simulink model "planta_CODESYS"  (R2025b)
settings: Solver=FixedStepAuto  StartTime=0.0  StopTime=inf  FixedStep=Ts2  MaxStep=1e-3  RelTol=1e-3
undefined symbols (not defined in the file): ah_max, at_max, bcx, bcy, bh_eq, bhb, bhEb, bhwu, bt, bt_eq, btb, btw, g, Hc, ih, it, Jh_eq, Jt_eq, Kcy, khwu, Ki_h, Ki_t, Kp_h, Kp_t, Ktw, lambda, Lh, Lh0, lh_0, Lt, magnitude, Mc_max, Ms, Mt, rhd, rtd, tau_hm, tau_tm, Thb_Max, ThEb_Max, Thm_0, Thm_Max, titahm_0, titatm_0, Ts0, Ts1, Ts2, Ttb_Max, Ttm_0, Ttm_Max, vh_0, vlx_0, vly_0, vt_0, vt_max, Wc, whm_0, whm_rated, wtm_0, xl_0 ... (+9)
libraries: simulink x10, opcualib x9, simulink_extras x2, dspnetwork x2, sl3dlib x1, hostiolib x1
(part 2 of 2)

== system planta_CODESYS/Controlador Izaje2 ==
  seleccion : Inport
  yh_enc : Inport  Port=2
  m_est : Inport  Port=3
  vh_lim : Inport  Port=4
  BRK_h : Inport  Port=5
  BRK_hE : Inport  Port=6
  vy_cmd : Inport  Port=7
  AND : Logic  IconShape=distinctive  AllPortsSameDT=off  OutDataTypeStr=boolean
  Controlador de Velocidad : MATLAB Function  TreatAsAtomicUnit=on
  Delay One Step : Delay  DelayLength=1  InitialCondition=Thm_0
  Modulación de la Referencia : MATLAB Function  TreatAsAtomicUnit=on
  Observador de Estado : MATLAB Function  TreatAsAtomicUnit=on
  vh_obs : Outport
  Thm_ref : Outport  Port=2
  wires:
  seleccion/1 -> Modulación de la Referencia/2(seleccion)
  m_est/1 -> Controlador de Velocidad/1(m_est)
  Delay One Step/1 -> Observador de Estado/2(Thm_ref)
  yh_enc/1 -> Observador de Estado/1(yh_enc)
  Observador de Estado/1(vh_obs) -> Controlador de Velocidad/3(vh_obs), vh_obs/1
  vy_cmd/1 -> Modulación de la Referencia/1(vy_cmd)
  Modulación de la Referencia/1(vh_ref) -> Controlador de Velocidad/2(vh_ref)
  AND/1 -> Controlador de Velocidad/4(BRK)
  BRK_hE/1 -> AND/2
  vh_lim/1 -> Modulación de la Referencia/3(vh_lim)
  BRK_h/1 -> AND/1
  Controlador de Velocidad/1(Thm_ref) -> Delay One Step/1, Thm_ref/1

== system planta_CODESYS/Modulador Carro ==
  Ttm_ref : Inport
  BRK_t : Inport  Port=2
  Constant1 : Constant  Value=0
  Gain2 : Gain  Gain=1/tau_tm
  Integrator : Integrator  InitialCondition=Ttm_0
  Saturation : Saturate  UpperLimit=Ttm_Max  LowerLimit=-Ttm_Max
  Sum : Sum  Inputs=|+-
  Switch : Switch  Criteria=u2 > Threshold  SaturateOnIntegerOverflow=off  InputSameDT=off
  Ttm : Outport
  wires:
  Saturation/1 -> Sum/1  "Ttm_lim"
  Sum/1 -> Gain2/1
  Gain2/1 -> Integrator/1
  Integrator/1 -> Ttm/1, Sum/2
  Ttm_ref/1 -> Switch/1
  BRK_t/1 -> Switch/2
  Switch/1 -> Saturation/1
  Constant1/1 -> Switch/3

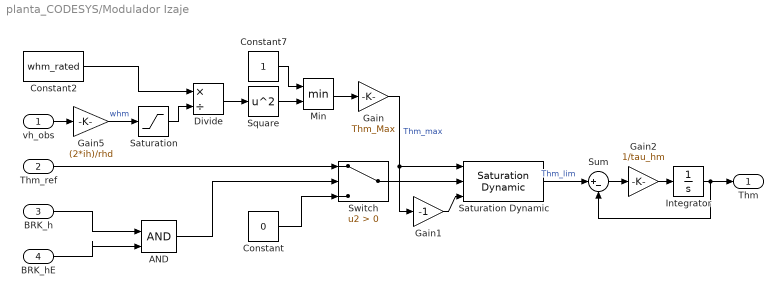
== system planta_CODESYS/Modulador Izaje ==
  vh_obs : Inport
  Thm_ref : Inport  Port=2
  BRK_h : Inport  Port=3
  BRK_hE : Inport  Port=4
  AND : Logic  IconShape=distinctive  AllPortsSameDT=off  OutDataTypeStr=boolean
  Constant : Constant  Value=0
  Constant2 : Constant  Value=whm_rated
  Constant7 : Constant
  Divide : Product  Inputs=*/
  Gain : Gain  Gain=Thm_Max
  Gain1 : Gain  Gain=-1
  Gain2 : Gain  Gain=1/tau_hm
  Gain5 : Gain  Gain=(2*ih)/rhd
  Integrator : Integrator  InitialCondition=Thm_0
  Min : MinMax  Inputs=2
  Saturation : Saturate  UpperLimit=inf  LowerLimit=whm_rated
  Saturation Dynamic : simulink/Discontinuities/Saturation Dynamic  OutMin=[]  OutMax=[]  OutDataTypeStr=Inherit: Same as second input  OutDataType=fixdt(1, 16)  OutScaling=2^-10  DoSatur=off
  Square : Math  Operator=square
  Sum : Sum  Inputs=|+-
  Switch : Switch  Criteria=u2 > Threshold  SaturateOnIntegerOverflow=off  InputSameDT=off
  Thm : Outport
  wires:
  Constant2/1 -> Divide/1
  Min/1 -> Gain/1
  Constant7/1 -> Min/1
  Gain/1 -> Gain1/1, Saturation Dynamic/1  "Thm_max"
  Saturation/1 -> Divide/2
  Square/1 -> Min/2
  Divide/1 -> Square/1
  vh_obs/1 -> Gain5/1
  Gain1/1 -> Saturation Dynamic/3
  Saturation Dynamic/1 -> Sum/1  "Thm_lim"
  Sum/1 -> Gain2/1
  Gain2/1 -> Integrator/1
  Integrator/1 -> Thm/1, Sum/2
  Thm_ref/1 -> Switch/1
  BRK_h/1 -> AND/1
  Switch/1 -> Saturation Dynamic/2
  BRK_hE/1 -> AND/2
  AND/1 -> Switch/2
  Gain5/1 -> Saturation/1  "whm"
  Constant/1 -> Switch/3

== system planta_CODESYS/Sensores Carro ==
  θtm : Inport
  xt : Inport  Port=2
  Encoder Carro : Subsystem
  Fines de carrera carro (rieles) : Subsystem
  xtd_enc : Outport
  FCE_izquierdo : Outport  Port=2
  FCE_derecho : Outport  Port=3
  FC_izquierdo : Outport  Port=4
  FC_derecho : Outport  Port=5
  wires:
  Fines de carrera carro (rieles)/1(FC_derecho) -> FC_derecho/1
  θtm/1 -> Encoder Carro/1(θtm)
  Fines de carrera carro (rieles)/2(FC_izquierdo) -> FC_izquierdo/1
  Fines de carrera carro (rieles)/3(FCE_derecho) -> FCE_derecho/1
  Fines de carrera carro (rieles)/4(FCE_izquierdo) -> FCE_izquierdo/1
  xt/1 -> Fines de carrera carro (rieles)/1(xt)
  Encoder Carro/1(xtd_enc) -> xtd_enc/1

== system planta_CODESYS/Sensores Izaje ==
  θhm : Inport
  Encoder Izaje : Subsystem
  Fines de carrera izaje (tambor) : Subsystem
  yh_enc : Outport
  FCE_inferior : Outport  Port=2
  FCE_superior : Outport  Port=3
  FC_inferior : Outport  Port=4
  FC_superior : Outport  Port=5
  wires:
  Fines de carrera izaje (tambor)/1(FC_superior) -> FC_superior/1
  Fines de carrera izaje (tambor)/4(FCE_inferior) -> FCE_inferior/1
  Fines de carrera izaje (tambor)/2(FC_inferior) -> FC_inferior/1
  Encoder Izaje/1(yh_enc) -> Fines de carrera izaje (tambor)/1(y_enc), yh_enc/1
  θhm/1 -> Encoder Izaje/1(θhm)
  Fines de carrera izaje (tambor)/3(FCE_superior) -> FCE_superior/1

== system planta_CODESYS/Subsistema Carro ==
  Fhw : Inport
  θl : Inport  Port=2
  Ttm : Inport  Port=3
  BRK_t : Inport  Port=4
  Accionamiento carro : Subsystem
  Dinámica carro : Subsystem
  Fuerza cable carro : Subsystem
  at : Outport
  vt : Outport  Port=2
  xt : Outport  Port=3
  θtm : Outport  Port=4
  wires:
  [Ftw] -> Accionamiento carro/1(Ftw)
  Accionamiento carro/1(θtm) -> θtm/1
  Dinámica carro/1(xt) -> Fuerza cable carro/3(xt), xt/1
  BRK_t/1 -> Accionamiento carro/3(BRK_t)
  [Ftw] -> Dinámica carro/1(Ftw)
  θl/1 -> Dinámica carro/2(θl)
  Ttm/1 -> Accionamiento carro/2(Ttm)
  Fuerza cable carro/1(Ftw) -> [Ftw]
  Dinámica carro/2(vt) -> Fuerza cable carro/4(vt), vt/1
  Accionamiento carro/2(xtd) -> Fuerza cable carro/1(xtd)
  Accionamiento carro/3(vtd) -> Fuerza cable carro/2(vtd)
  Fhw/1 -> Dinámica carro/3(Fhw)
  Dinámica carro/3(at) -> at/1

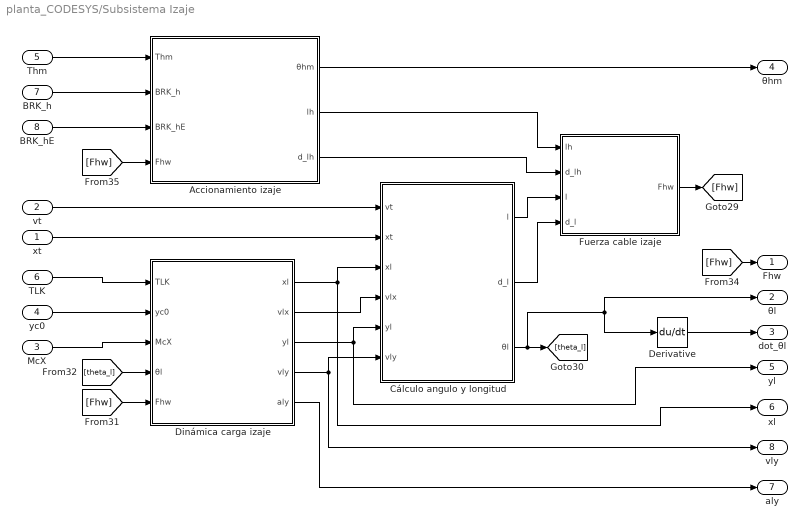
== system planta_CODESYS/Subsistema Izaje ==
  xt : Inport
  vt : Inport  Port=2
  McX : Inport  Port=3
  yc0 : Inport  Port=4
  Thm : Inport  Port=5
  TLK : Inport  Port=6
  BRK_h : Inport  Port=7
  BRK_hE : Inport  Port=8
  Accionamiento izaje : Subsystem
  Cálculo angulo y longitud : Subsystem
  Derivative : Derivative
  Dinámica carga izaje : Subsystem
  Fuerza cable izaje : Subsystem
  Fhw : Outport
  θl : Outport  Port=2
  dot_θl : Outport  Port=3
  θhm : Outport  Port=4
  yl : Outport  Port=5
  xl : Outport  Port=6
  aly : Outport  Port=7
  vly : Outport  Port=8
  wires:
  vt/1 -> Cálculo angulo y longitud/1(vt)
  Accionamiento izaje/2(lh) -> Fuerza cable izaje/1(lh)
  yc0/1 -> Dinámica carga izaje/2(yc0)
  McX/1 -> Dinámica carga izaje/3(McX)
  Dinámica carga izaje/4(vly) -> vly/1, Cálculo angulo y longitud/6(vly)
  [Fhw] -> Accionamiento izaje/4(Fhw)
  [theta_l] -> Dinámica carga izaje/4(θl)
  xt/1 -> Cálculo angulo y longitud/2(xt)
  BRK_h/1 -> Accionamiento izaje/2(BRK_h)
  Dinámica carga izaje/1(xl) -> Cálculo angulo y longitud/3(xl), xl/1
  Dinámica carga izaje/2(vlx) -> Cálculo angulo y longitud/4(vlx)
  Fuerza cable izaje/1(Fhw) -> [Fhw]
  Cálculo angulo y longitud/1(l) -> Fuerza cable izaje/3(l)
  Accionamiento izaje/1(θhm) -> θhm/1
  Cálculo angulo y longitud/3(θl) -> θl/1, Derivative/1, [theta_l]
  TLK/1 -> Dinámica carga izaje/1(TLK)
  [Fhw] -> Dinámica carga izaje/5(Fhw)
  BRK_hE/1 -> Accionamiento izaje/3(BRK_hE)
  Thm/1 -> Accionamiento izaje/1(Thm)
  Dinámica carga izaje/3(yl) -> Cálculo angulo y longitud/5(yl), yl/1
  Cálculo angulo y longitud/2(d_l) -> Fuerza cable izaje/4(d_l)
  Accionamiento izaje/3(d_lh) -> Fuerza cable izaje/2(d_lh)
  Dinámica carga izaje/5(aly) -> aly/1
  [Fhw] -> Fhw/1
  Derivative/1 -> dot_θl/1

== system planta_CODESYS/Sensores Carro/Encoder Carro ==
  θtm : Inport
  Gain1 : Gain  Gain=rtd/it
  xtd_enc : Outport
  wires:
  θtm/1 -> Gain1/1
  Gain1/1 -> xtd_enc/1

== system planta_CODESYS/Sensores Carro/Fines de carrera carro (rieles) ==
  xt : Inport
  Compare To Constant : simulink/Logic and Bit Operations/Compare To Constant  relop=>=  const=xt_max  OutDataTypeStr=boolean
  Compare To Constant1 : simulink/Logic and Bit Operations/Compare To Constant  relop=>=  const=xt_max+0.5  OutDataTypeStr=boolean
  Compare To Constant2 : simulink/Logic and Bit Operations/Compare To Constant  relop=<=  const=xt_min  OutDataTypeStr=boolean
  Compare To Constant3 : simulink/Logic and Bit Operations/Compare To Constant  relop=<=  const=xt_min-0.5  OutDataTypeStr=boolean
  FC_derecho : Outport
  FC_izquierdo : Outport  Port=2
  FCE_derecho : Outport  Port=3
  FCE_izquierdo : Outport  Port=4
  wires:
  Compare To Constant2/1 -> FC_izquierdo/1
  xt/1 -> Compare To Constant/1, Compare To Constant1/1, Compare To Constant2/1, Compare To Constant3/1
  Compare To Constant3/1 -> FCE_izquierdo/1
  Compare To Constant1/1 -> FCE_derecho/1
  Compare To Constant/1 -> FC_derecho/1

== system planta_CODESYS/Sensores Izaje/Encoder Izaje ==
  θhm : Inport
  Gain3 : Gain  Gain=rhd/(2*ih)
  yh_enc : Outport
  wires:
  θhm/1 -> Gain3/1
  Gain3/1 -> yh_enc/1

== system planta_CODESYS/Sensores Izaje/Fines de carrera izaje (tambor) ==
  y_enc : Inport
  Compare To Constant4 : simulink/Logic and Bit Operations/Compare To Constant  relop=>=  const=yh_max  OutDataTypeStr=boolean
  Compare To Constant5 : simulink/Logic and Bit Operations/Compare To Constant  relop=>=  const=yh_max+0.5  OutDataTypeStr=boolean
  Compare To Constant6 : simulink/Logic and Bit Operations/Compare To Constant  relop=<=  const=yh_min  OutDataTypeStr=boolean
  Compare To Constant7 : simulink/Logic and Bit Operations/Compare To Constant  relop=<=  const=yh_min-0.5  OutDataTypeStr=boolean
  FC_superior : Outport
  FC_inferior : Outport  Port=2
  FCE_superior : Outport  Port=3
  FCE_inferior : Outport  Port=4
  wires:
  Compare To Constant7/1 -> FCE_inferior/1
  y_enc/1 -> Compare To Constant7/1, Compare To Constant6/1, Compare To Constant4/1, Compare To Constant5/1
  Compare To Constant6/1 -> FC_inferior/1
  Compare To Constant5/1 -> FCE_superior/1
  Compare To Constant4/1 -> FC_superior/1

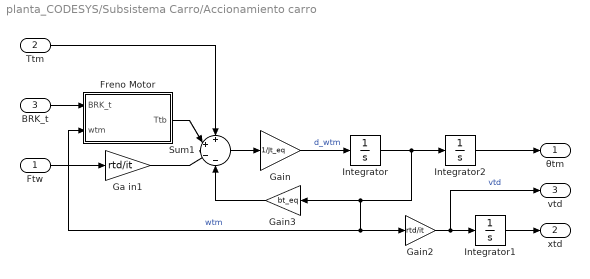
== system planta_CODESYS/Subsistema Carro/Accionamiento carro ==
  Ftw : Inport
  Ttm : Inport  Port=2
  BRK_t : Inport  Port=3
  Freno Motor : Subsystem
  Ga in1 : Gain  Gain=rtd/it
  Gain : Gain  Gain=1/Jt_eq
  Gain2 : Gain  Gain=rtd/it
  Gain3 : Gain  Gain=bt_eq
  Integrator : Integrator  InitialCondition=wtm_0
  Integrator1 : Integrator  InitialCondition=xtd_0
  Integrator2 : Integrator  InitialCondition=titatm_0
  Sum1 : Sum  Inputs=++--
  θtm : Outport
  xtd : Outport  Port=2
  vtd : Outport  Port=3
  wires:
  Sum1/1 -> Gain/1
  Integrator/1 -> Gain2/1, Freno Motor/2(wtm), Gain3/1, Integrator2/1  "wtm"
  Gain2/1 -> Integrator1/1, vtd/1  "vtd"
  Ttm/1 -> Sum1/1
  Gain/1 -> Integrator/1  "d_wtm"
  BRK_t/1 -> Freno Motor/1(BRK_t)
  Integrator1/1 -> xtd/1
  Ftw/1 -> Ga in1/1
  Ga in1/1 -> Sum1/3
  Freno Motor/1(Ttb) -> Sum1/2
  Gain3/1 -> Sum1/4
  Integrator2/1 -> θtm/1

== system planta_CODESYS/Subsistema Carro/Dinámica carro ==
  Ftw : Inport
  θl : Inport  Port=2
  Fhw : Inport  Port=3
  Gain : Gain  Gain=2
  Gain1 : Gain  Gain=1/Mt
  Gain2 : Gain  Gain=bt
  Integrator : Integrator  InitialCondition=vt_0
  Integrator1 : Integrator  InitialCondition=xt_0
  Product : Product
  Sin : Trigonometry
  Sum : Sum  Inputs=++-
  xt : Outport
  vt : Outport  Port=2
  at : Outport  Port=3
  wires:
  Gain1/1 -> at/1, Integrator/1  "dot_vt"
  Integrator/1 -> Gain2/1, vt/1, Integrator1/1  "vt"
  Gain2/1 -> Sum/3
  Sum/1 -> Gain1/1
  Integrator1/1 -> xt/1  "xt"
  Fhw/1 -> Gain/1
  Gain/1 -> Product/2
  θl/1 -> Sin/1
  Sin/1 -> Product/1
  Product/1 -> Sum/2  "F_coupling"
  Ftw/1 -> Sum/1

== system planta_CODESYS/Subsistema Carro/Fuerza cable carro ==
  xtd : Inport
  vtd : Inport  Port=2
  xt : Inport  Port=3
  vt : Inport  Port=4
  Gain : Gain  Gain=Ktw
  Gain1 : Gain  Gain=btw
  Sum : Sum  Inputs=+-
  Sum1 : Sum
  Sum2 : Sum  Inputs=+-
  Ftw : Outport
  wires:
  xtd/1 -> Sum/1
  Gain1/1 -> Sum1/2
  Sum/1 -> Gain/1
  xt/1 -> Sum/2
  Sum2/1 -> Gain1/1
  Gain/1 -> Sum1/1
  vt/1 -> Sum2/2
  Sum1/1 -> Ftw/1  "Ftw"
  vtd/1 -> Sum2/1

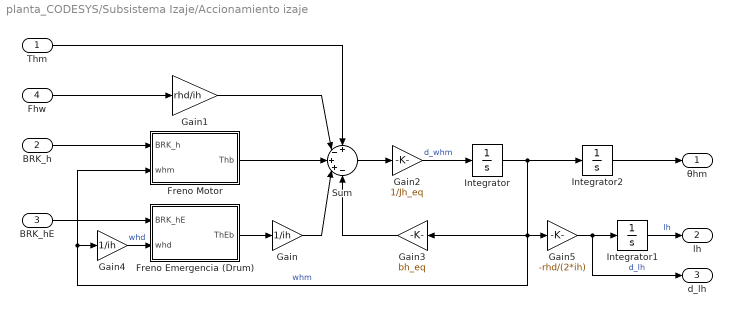
== system planta_CODESYS/Subsistema Izaje/Accionamiento izaje ==
  Thm : Inport
  BRK_h : Inport  Port=2
  BRK_hE : Inport  Port=3
  Fhw : Inport  Port=4
  Freno Emergencia (Drum) : Subsystem
  Freno Motor : Subsystem
  Gain : Gain  Gain=1/ih
  Gain1 : Gain  Gain=rhd/ih
  Gain2 : Gain  Gain=1/Jh_eq
  Gain3 : Gain  Gain=bh_eq
  Gain4 : Gain  Gain=1/ih
  Gain5 : Gain  Gain=-rhd/(2*ih)
  Integrator : Integrator  InitialCondition=whm_0
  Integrator1 : Integrator  InitialCondition=lh_0
  Integrator2 : Integrator  InitialCondition=titahm_0
  Sum : Sum  Inputs=+-++-
  θhm : Outport
  lh : Outport  Port=2
  d_lh : Outport  Port=3
  wires:
  Gain5/1 -> d_lh/1, Integrator1/1  "d_lh"
  Integrator/1 -> Gain3/1, Freno Motor/2(whm), Gain4/1, Gain5/1, Integrator2/1  "whm"
  Freno Emergencia (Drum)/1(ThEb) -> Gain/1
  Gain3/1 -> Sum/5
  BRK_h/1 -> Freno Motor/1(BRK_h)
  Gain/1 -> Sum/4
  Gain2/1 -> Integrator/1  "d_whm"
  Sum/1 -> Gain2/1
  Gain4/1 -> Freno Emergencia (Drum)/2(whd)  "whd"
  BRK_hE/1 -> Freno Emergencia (Drum)/1(BRK_hE)
  Fhw/1 -> Gain1/1
  Freno Motor/1(Thb) -> Sum/3
  Gain1/1 -> Sum/2
  Integrator1/1 -> lh/1  "lh"
  Integrator2/1 -> θhm/1
  Thm/1 -> Sum/1

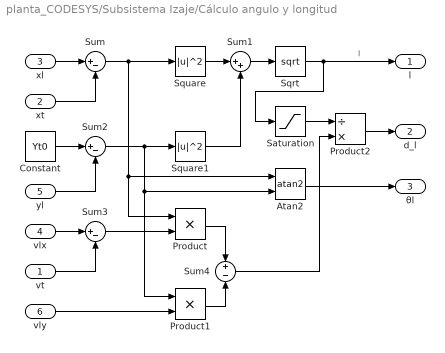
== system planta_CODESYS/Subsistema Izaje/Cálculo angulo y longitud ==
  vt : Inport
  xt : Inport  Port=2
  xl : Inport  Port=3
  vlx : Inport  Port=4
  yl : Inport  Port=5
  vly : Inport  Port=6
  Atan2 : Trigonometry  Operator=atan2
  Constant : Constant  Value=Yt0
  Product : Product
  Product1 : Product
  Product2 : Product  Inputs=/*
  Saturation : Saturate  UpperLimit=inf  LowerLimit=0.1
  Sqrt : Sqrt
  Square : Math  Operator=magnitude^2
  Square1 : Math  Operator=magnitude^2
  Sum : Sum  Inputs=|+-
  Sum1 : Sum  Inputs=|++
  Sum2 : Sum  Inputs=|+-
  Sum3 : Sum  Inputs=|+-
  Sum4 : Sum  Inputs=+-
  l : Outport
  d_l : Outport  Port=2
  θl : Outport  Port=3
  wires:
  Product2/1 -> d_l/1
  Sqrt/1 -> l/1, Saturation/1  "l"
  Sum1/1 -> Sqrt/1
  Sum2/1 -> Product1/1, Atan2/2, Square1/1
  Sum/1 -> Product/1, Atan2/1, Square/1
  yl/1 -> Sum2/2
  Atan2/1 -> θl/1
  vly/1 -> Product1/2
  xl/1 -> Sum/1
  Constant/1 -> Sum2/1
  Sum3/1 -> Product/2
  Square1/1 -> Sum1/2
  vt/1 -> Sum3/2
  Sum4/1 -> Product2/2
  vlx/1 -> Sum3/1
  xt/1 -> Sum/2
  Square/1 -> Sum1/1
  Product1/1 -> Sum4/2
  Product/1 -> Sum4/1
  Saturation/1 -> Product2/1

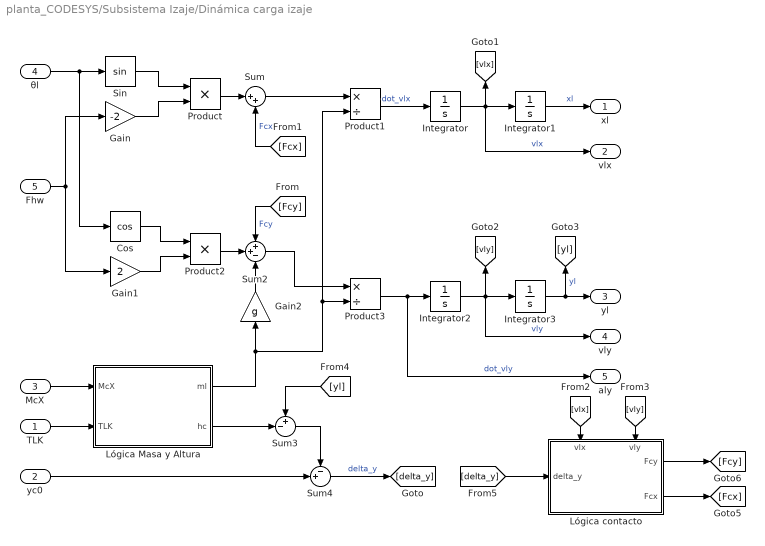
== system planta_CODESYS/Subsistema Izaje/Dinámica carga izaje ==
  TLK : Inport
  yc0 : Inport  Port=2
  McX : Inport  Port=3
  θl : Inport  Port=4
  Fhw : Inport  Port=5
  Cos : Trigonometry  Operator=cos
  Gain : Gain  Gain=-2
  Gain1 : Gain  Gain=2
  Gain2 : Gain  Gain=g
  Integrator : Integrator  InitialCondition=vlx_0
  Integrator1 : Integrator  InitialCondition=xl_0
  Integrator2 : Integrator  InitialCondition=vly_0
  Integrator3 : Integrator  InitialCondition=yl_0
  Lógica Masa y Altura : Subsystem
  Lógica contacto : Subsystem
      settings: PortSchema="{\"entries\":[{\"content\":{\"sides\":[{\"content\":{\"connectorIds\":[\"In1\"]},\"type\":\"ConnectorPlacement.EquallySpacedRectSide\",\"uuid\":\"20a8b2c4-d5cf-44ce-93ec-929b996a0905\"},{\"content\":{\"connectorIds\":[\"Out1\",\"Out2\"],\"side\":\"RIGHT\"},\"type\":\"ConnectorPlacement.EquallySpacedRectSide\",\"uuid\":\"396e1f2e-cf71-48dc-8d57-a3e2695dfff1\"},{\"content\":{\"connectorIds\":[\"In2\",\"In3\"],\"side\":\"TOP\"},\"type\":\"ConnectorPlacement.EquallySpacedRectSide\",\"uuid\":\"e66c0478-9682-41e1-9b77-d2d789a9c323\"}]},\"type\":\"ConnectorPlacement.EquallySpacedConnector\",\"uuid\":\"193dabd2-f524-433a-b6ef-c1cab585578e\"}],\"packageUris\":[\"http://schema.mathworks.com/mf0/Connector/R2020b\"],\"version\":\"1.0\"}"
  Product : Product
  Product1 : Product  Inputs=*/
  Product2 : Product
  Product3 : Product  Inputs=*/
  Sin : Trigonometry
  Sum : Sum  Inputs=|++
  Sum2 : Sum  Inputs=++-
  Sum3 : Sum  Inputs=+-|
  Sum4 : Sum  Inputs=-+|
  xl : Outport
  vlx : Outport  Port=2
  yl : Outport  Port=3
  vly : Outport  Port=4
  aly : Outport  Port=5
  wires:
  θl/1 -> Sin/1, Cos/1
  Integrator/1 -> vlx/1, Integrator1/1, [vlx]  "vlx"
  Sum3/1 -> Sum4/1
  Sin/1 -> Product/1
  Gain/1 -> Product/2
  [Fcy] -> Sum2/1  "Fcy"
  Integrator2/1 -> vly/1, Integrator3/1, [vly]  "vly"
  Integrator3/1 -> yl/1, [yl]  "yl"
  Fhw/1 -> Gain1/1, Gain/1
  [Fcx] -> Sum/2  "Fcx"
  Product/1 -> Sum/1
  Product1/1 -> Integrator/1  "dot_vlx"
  Gain2/1 -> Sum2/3
  Cos/1 -> Product2/1
  Gain1/1 -> Product2/2
  [yl] -> Sum3/1
  Product2/1 -> Sum2/2
  yc0/1 -> Sum4/2
  Sum2/1 -> Product3/1
  Product3/1 -> aly/1, Integrator2/1  "dot_vly"
  Sum/1 -> Product1/1
  Integrator1/1 -> xl/1  "xl"
  Sum4/1 -> [delta_y]  "delta_y"
  Lógica contacto/1(Fcy) -> [Fcy]
  Lógica contacto/2(Fcx) -> [Fcx]
  Lógica Masa y Altura/1(ml) -> Product1/2, Product3/2, Gain2/1
  McX/1 -> Lógica Masa y Altura/1(McX)
  TLK/1 -> Lógica Masa y Altura/2(TLK)
  Lógica Masa y Altura/2(hc) -> Sum3/2
  [vlx] -> Lógica contacto/2(vlx)
  [vly] -> Lógica contacto/3(vly)
  [delta_y] -> Lógica contacto/1(delta_y)

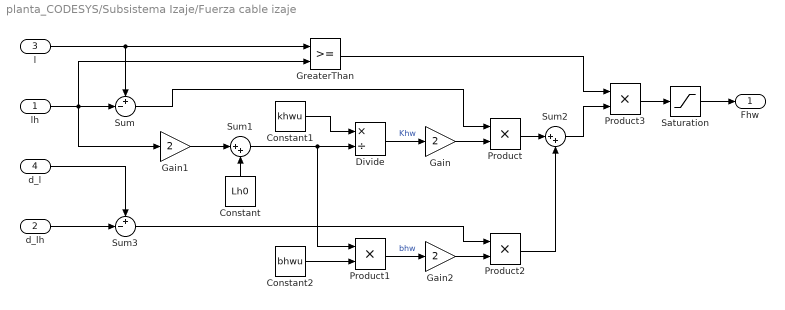
== system planta_CODESYS/Subsistema Izaje/Fuerza cable izaje ==
  lh : Inport
  d_lh : Inport  Port=2
  l : Inport  Port=3
  d_l : Inport  Port=4
  Constant : Constant  Value=Lh0
  Constant1 : Constant  Value=khwu
  Constant2 : Constant  Value=bhwu
  Divide : Product  Inputs=*/  RndMeth=Zero  SaturateOnIntegerOverflow=on
  Gain : Gain  Gain=2
  Gain1 : Gain  Gain=2
  Gain2 : Gain  Gain=2
  GreaterThan : RelationalOperator  OutDataTypeStr=boolean  RndMeth=Simplest  InputSameDT=off
  Product{,1..3} (4 alike) : Product
  Saturation : Saturate  UpperLimit=inf  LowerLimit=0
  Sum : Sum  Inputs=+-|
  Sum1 : Sum  Inputs=|++
  Sum2 : Sum  Inputs=|++
  Sum3 : Sum  Inputs=+-|
  Fhw : Outport
  wires:
  Constant/1 -> Sum1/2
  Constant2/1 -> Product1/2
  Sum1/1 -> Divide/2, Product1/1
  lh/1 -> Sum/2, GreaterThan/2, Gain1/1
  Product/1 -> Sum2/1
  Gain1/1 -> Sum1/1
  l/1 -> Sum/1, GreaterThan/1
  Product2/1 -> Sum2/2
  Product3/1 -> Saturation/1
  GreaterThan/1 -> Product3/1
  d_lh/1 -> Sum3/2
  Constant1/1 -> Divide/1
  Product1/1 -> Gain2/1  "bhw"
  Sum/1 -> Product/1
  Gain2/1 -> Product2/2
  Divide/1 -> Gain/1  "Khw"
  Sum2/1 -> Product3/2
  Sum3/1 -> Product2/1
  d_l/1 -> Sum3/1
  Gain/1 -> Product/2
  Saturation/1 -> Fhw/1

== system planta_CODESYS/Subsistema Carro/Accionamiento carro/Freno Motor ==
  BRK_t : Inport
  wtm : Inport  Port=2
  Constant : Constant  Value=0
  Gain3 : Gain  Gain=-Ttb_Max
  Gain4 : Gain  Gain=btb
  Switch : Switch  Criteria=u2 > Threshold  SaturateOnIntegerOverflow=off  InputSameDT=off
  Tanh : Trigonometry  Operator=tanh
  Ttb : Outport
  wires:
  BRK_t/1 -> Switch/2
  Constant/1 -> Switch/1
  wtm/1 -> Gain4/1
  Gain4/1 -> Tanh/1
  Tanh/1 -> Gain3/1
  Gain3/1 -> Switch/3
  Switch/1 -> Ttb/1

== system planta_CODESYS/Subsistema Izaje/Accionamiento izaje/Freno Emergencia (Drum) ==
  BRK_hE : Inport
  whd : Inport  Port=2
  Constant : Constant  Value=0
  Gain3 : Gain  Gain=-ThEb_Max
  Gain4 : Gain  Gain=bhEb
  Switch : Switch  Criteria=u2 > Threshold  SaturateOnIntegerOverflow=off  InputSameDT=off
  Tanh : Trigonometry  Operator=tanh
  ThEb : Outport
  wires:
  BRK_hE/1 -> Switch/2
  Gain3/1 -> Switch/3
  Constant/1 -> Switch/1
  whd/1 -> Gain4/1
  Gain4/1 -> Tanh/1
  Tanh/1 -> Gain3/1
  Switch/1 -> ThEb/1

== system planta_CODESYS/Subsistema Izaje/Accionamiento izaje/Freno Motor ==
  BRK_h : Inport
  whm : Inport  Port=2
  Constant : Constant  Value=0
  Gain3 : Gain  Gain=-Thb_Max
  Gain4 : Gain  Gain=bhb
  Switch : Switch  Criteria=u2 > Threshold  SaturateOnIntegerOverflow=off  InputSameDT=off
  Tanh : Trigonometry  Operator=tanh
  Thb : Outport
  wires:
  BRK_h/1 -> Switch/2
  Gain3/1 -> Switch/3
  Constant/1 -> Switch/1
  whm/1 -> Gain4/1
  Gain4/1 -> Tanh/1
  Tanh/1 -> Gain3/1
  Switch/1 -> Thb/1

== system planta_CODESYS/Subsistema Izaje/Dinámica carga izaje/Lógica Masa y Altura ==
  McX : Inport
  TLK : Inport  Port=2
  Constant : Constant  Value=Ms
  Constant1 : Constant  Value=0
  Constant2 : Constant  Value=Hc
  Rate Limiter : RateLimiter  Commented=through  RisingSlewLimit=Mc_max/0.1  FallingSlewLimit=-Mc_max/0.1  SampleTimeMode=inherited  InitialCondition=Ms
  Sum1 : Sum  Inputs=|++
  Switch : Switch  Criteria=u2 > Threshold  SaturateOnIntegerOverflow=off  InputSameDT=off
  Switch1 : Switch  Criteria=u2 > Threshold  SaturateOnIntegerOverflow=off  InputSameDT=off
  ml : Outport
  hc : Outport  Port=2
  wires:
  Sum1/1 -> Switch/1
  Constant2/1 -> Switch1/1
  TLK/1 -> Switch1/2, Switch/2
  Constant/1 -> Switch/3, Sum1/2
  Constant1/1 -> Switch1/3
  McX/1 -> Sum1/1
  Switch/1 -> Rate Limiter/1
  Rate Limiter/1 -> ml/1
  Switch1/1 -> hc/1

== system planta_CODESYS/Subsistema Izaje/Dinámica carga izaje/Lógica contacto ==
  delta_y : Inport
  vlx : Inport  Port=2
  vly : Inport  Port=3
  Constant3 : Constant  Value=0
  Constant4 : Constant  Value=0
  Gain3 : Gain  Gain=Kcy
  Gain4 : Gain  Gain=bcy
  Gain5 : Gain  Gain=-bcx
  Saturation : Saturate  UpperLimit=60e5  LowerLimit=0
  Sum5 : Sum  Inputs=-+|
  Switch2 : Switch  SaturateOnIntegerOverflow=off  InputSameDT=off
  Switch3 : Switch  SaturateOnIntegerOverflow=off  InputSameDT=off
  Fcy : Outport
  Fcx : Outport  Port=2
  wires:
  Sum5/1 -> Switch2/1
  vlx/1 -> Gain5/1
  Gain4/1 -> Sum5/1
  vly/1 -> Gain4/1
  Constant4/1 -> Switch3/3
  Gain5/1 -> Switch3/1
  Gain3/1 -> Sum5/2
  delta_y/1 -> Switch3/2, Gain3/1, Switch2/2
  Constant3/1 -> Switch2/3
  Switch2/1 -> Saturation/1  "Fcy"
  Switch3/1 -> Fcx/1  "Fcx"
  Saturation/1 -> Fcy/1

== matlab function planta_CODESYS/Controlador Izaje2/Controlador de Velocidad ==
  data: m_est input; Thm_ref output; vh_ref input; vh_obs input; BRK input; ih parameter; rhd parameter; g parameter; Kp_h parameter; Ki_h parameter; Ts2 parameter
function Thm_ref = ControlVelocidad(m_est, vh_ref, vh_obs, BRK, ih, rhd, g, Kp_h, Ki_h, Ts2)
persistent int_prev e_w_prev

if isempty(int_prev)
    int_prev = 0.0;
    e_w_prev = 0.0;
end

e_w = (vh_ref - vh_obs) * (2 * ih / rhd);

if BRK > 0
    int_val = int_prev + (Ts2 / 2) * (e_w + e_w_prev);
else
    int_val = 0.0;
    e_w_prev = 0.0;
end

T_PID = Kp_h * e_w + Ki_h * int_val;
Tg_ff = m_est * (g * rhd / (2 * ih));

Thm_ref = T_PID + Tg_ff;

int_prev = int_val;
e_w_prev = e_w;
end

== matlab function planta_CODESYS/Controlador Izaje2/Observador de Estado ==
  data: yh_enc input; vh_obs output; Thm_ref input; whm_0 parameter; titahm_0 parameter; Lh parameter; bh_eq parameter; Jh_eq parameter; rhd parameter; ih parameter; Ts2 parameter; Ms parameter; g parameter
function vh_obs = Observador_Estado_h(yh_enc, Thm_ref, whm_0, titahm_0,...
    Lh, bh_eq, Jh_eq, rhd, ih, Ts2, Ms, g)
    
    % Memorias
    persistent theta_h_obs_prev wh_obs_prev int_e_prev
    
    % Condiciones iniciales
    if isempty(theta_h_obs_prev)
        theta_h_obs_prev = titahm_0;
        wh_obs_prev      = whm_0;    
        int_e_prev       = 0.0; 
    end
    
    % 1. Convertir posición lineal del carro a angular del motor
    theta_h_enc = yh_enc * (2*ih / rhd);
    
    % 2. Error de estimación (Posición real vs observada)
    e_theta_h = theta_h_enc - theta_h_obs_prev;
    
    % 3. Lazo de torque (Física de la planta)
    Torque_net = Thm_ref - (Ms*g*rhd/(2*ih)) - (bh_eq * wh_obs_prev) +...
        (Lh(3) * int_e_prev);
    alpha_phys = Torque_net / Jh_eq; % Aceleración angular
    
    % 4. Derivadas
    dot_wh_obs      = alpha_phys + (Lh(2) * e_theta_h);
    dot_theta_h_obs = wh_obs_prev + (Lh(1) * e_theta_h);

    % 5. Salida del observador
    vh_obs = wh_obs_prev * (rhd / (2*ih));
    
    % 6. Integración Discreta
    theta_h_obs = theta_h_obs_prev + (Ts2 * dot_theta_h_obs);
    wh_obs      = wh_obs_prev      + (Ts2 * dot_wh_obs);
    int_e       = int_e_prev       + (Ts2 * e_theta_h);

    % 7. Actualizar memorias para el siguiente ciclo de reloj
    theta_h_obs_prev = theta_h_obs;
    wh_obs_prev      = wh_obs;
    int_e_prev       = int_e;
end

== matlab function planta_CODESYS/MATLAB Function2 ==
  data: TLK input; M_carga output; Mc_min parameter
function M_carga = Masa_Aleatoria(TLK, Mc_min)
    persistent masa_actual;
    persistent ultimo_estado_trigger;
    
    % Inicialización
    if isempty(masa_actual)
        masa_actual = Mc_min; % Empezamos con el valor mínimo por defecto
        ultimo_estado_trigger = 0;
    end
    
    % DETECCIÓN DE FLANCO DE SUBIDA (Rising Edge)
    if (TLK == 1 && ultimo_estado_trigger == 0)
        % Generar carga aleatoria entre 3tn y 55tn (para tener sobrecarga)
        masa_actual = Mc_min + (55000 - Mc_min) * rand();
        masa_actual = round(masa_actual); 
    end
    
    % Actualizar memoria del trigger
    ultimo_estado_trigger = TLK;
    % Salida: La masa se mantiene constante hasta el próximo trigger
    M_carga = masa_actual;
end

== matlab function planta_CODESYS/MATLAB Function3 ==
  data: yc0 output; xl input; xt_min parameter; Wc parameter; h_vec input
function yc0 = Y_spreader(xl, xt_min, Wc, h_vec)
% Cálculo índice de spreader
i_spreader = floor((xl - xt_min)/Wc) + 1;
i_spreader = min(max(i_spreader, 1), 33);

% Obtención de yc0 usando la posición del spreader
yc0 = h_vec(i_spreader);

== matlab function planta_CODESYS/Controlador Carro2/Controlador de Balanceo ==
  data: tita_l input; v_sway output; yh_enc input; anti_sway input; Yt0 parameter; g parameter; lambda parameter
function v_sway = ControlBalanceo(tita_l, yh_enc, anti_sway, Yt0, g, lambda)

lh = abs(Yt0 - yh_enc);

K_sway = 2 * lambda * sqrt(g*lh);

if(anti_sway)
    v_sway = K_sway * tita_l;
else
    v_sway = 0;
end

== matlab function planta_CODESYS/Controlador Carro2/Modulación de la Referencia ==
  data: vx_cmd input; seleccion input; vt_ref output; v_sway input; Ts2 parameter; at_max parameter; vt_max parameter; vt_0 parameter
function vt_ref = ModulacionRef(vx_cmd, seleccion, v_sway, Ts2, at_max, vt_max, vt_0)

persistent vt_ref_prev

if isempty(vt_ref_prev)
    vt_ref_prev = vt_0;
end

if seleccion > 0
    vel_base = 0;
else
    vel_base = vx_cmd;
end

vt_cmd = vel_base + v_sway;
vt_cmd_sat = min(max(vt_cmd, -vt_max), vt_max);

delta_v = vt_cmd_sat - vt_ref_prev;
limite_delta = at_max * Ts2;
delta_v_limitado = min(max(delta_v, -limite_delta), limite_delta);

vt_ref = vt_ref_prev + delta_v_limitado;
vt_ref_prev = vt_ref;

== matlab function planta_CODESYS/Controlador Carro2/Observador de Estado ==
  data: xtd_enc input; vt_obs output; Ttm_ref input; wtm_0 parameter; titatm_0 parameter; Lt parameter; bt_eq parameter; Jt_eq parameter; rtd parameter; it parameter; Ts2 parameter
function vt_obs = Observador_Estado_t(xtd_enc, Ttm_ref, wtm_0, titatm_0, Lt, bt_eq, Jt_eq, rtd, it, Ts2)...
    
    % Memorias
    persistent theta_t_obs_prev wt_obs_prev int_e_prev
    
    % Condiciones iniciales
    if isempty(theta_t_obs_prev)
        theta_t_obs_prev = titatm_0;
        wt_obs_prev      = wtm_0;    
        int_e_prev       = 0.0; 
    end
    
    % 1. Convertir posición lineal del carro a angular del motor
    theta_t_enc = xtd_enc * (it / rtd);
    
    % 2. Error de estimación (Posición real vs observada)
    e_theta_t = theta_t_enc - theta_t_obs_prev;
    
    % 3. Lazo de torque (Física de la planta)
    Torque_net = Ttm_ref - (bt_eq * wt_obs_prev) + (Lt(3) * int_e_prev);
    alpha_phys = Torque_net / Jt_eq; % Aceleración angular
    
    % 4. Derivadas
    dot_wt_obs      = alpha_phys + (Lt(2) * e_theta_t);
    dot_theta_t_obs = wt_obs_prev + (Lt(1) * e_theta_t);

    % 5. Salida del observador
    vt_obs = wt_obs_prev * (rtd / it);
    
    % 6. Integración Discreta
    theta_t_obs = theta_t_obs_prev + (Ts2 * dot_theta_t_obs);
    wt_obs      = wt_obs_prev      + (Ts2 * dot_wt_obs);
    int_e       = int_e_prev       + (Ts2 * e_theta_t);

    % 7. Actualizar memorias para el siguiente ciclo de reloj
    theta_t_obs_prev = theta_t_obs;
    wt_obs_prev      = wt_obs;
    int_e_prev       = int_e;
end

== matlab function planta_CODESYS/Controlador Carro2/Controlador de Velocidad ==
  data: vt_ref input; Ttm_ref output; vt_obs input; BRK_t input; Ts2 parameter; Ki_t parameter; Kp_t parameter
function Ttm_ref = ControlVelocidad(vt_ref, vt_obs, BRK_t, Ts2, Ki_t, Kp_t)
    % Memorias para el integrador
    persistent int_prev e_v_prev
    
    % Inicialización
    if isempty(int_prev)
        int_prev = 0.0;
        e_v_prev = 0.0;
    end
    
    % 1. Cálculo del error de velocidad
    e_v = vt_ref - vt_obs;
    
    % 2. Integrador Discreto (Tustin) con Reset por Freno
    % Si el freno está activo (BRK_t = 0), forzamos la memoria a 0 
    % para evitar la acumulación de error (Anti-Windup).
    if BRK_t > 0
        int_val = int_prev + (Ts2 / 2) * (e_v + e_v_prev);
    else
        int_val = 0.0;
    end
    
    % 3. Controlador PI
    P_out = e_v * Kp_t;
    I_out = int_val * Ki_t;
    
    % Suma final de referencia de torque
    Ttm_ref = P_out + I_out;
    
    % 4. Actualizar memorias
    int_prev = int_val;
    e_v_prev = e_v;
end

== matlab function planta_CODESYS/Controlador Izaje2/Modulación de la Referencia ==
  data: vy_cmd input; vh_ref output; seleccion input; ah_max parameter; Ts2 parameter; vh_0 parameter; vh_lim input
function vh_ref = ModulacionReferencia(vy_cmd, seleccion, ah_max, Ts2, vh_0, vh_lim)
persistent vh_ref_prev

if isempty(vh_ref_prev)
    vh_ref_prev = vh_0;
end

if seleccion > 0
    vh_cmd = 0;
else
    vh_cmd = vy_cmd;
end

vh_cmd_sat = min(max(vh_cmd, -vh_lim), vh_lim);

delta_v = vh_cmd_sat - vh_ref_prev;
limite_delta = ah_max * Ts2;
delta_v_limitado = min(max(delta_v, -limite_delta), limite_delta);

vh_ref = vh_ref_prev + delta_v_limitado;
vh_ref_prev = vh_ref;
end
